simulink model "oven"  (Simulink 7.4)
settings: Solver=ode45  StartTime=0.0  StopTime=1000  MaxStep=0.1  RelTol=1e-3
undefined symbols (not defined in the file): slDataTypeAndScale
libraries: simulink x1
settings Model: Creator=psonna  LastModifiedBy=psonna

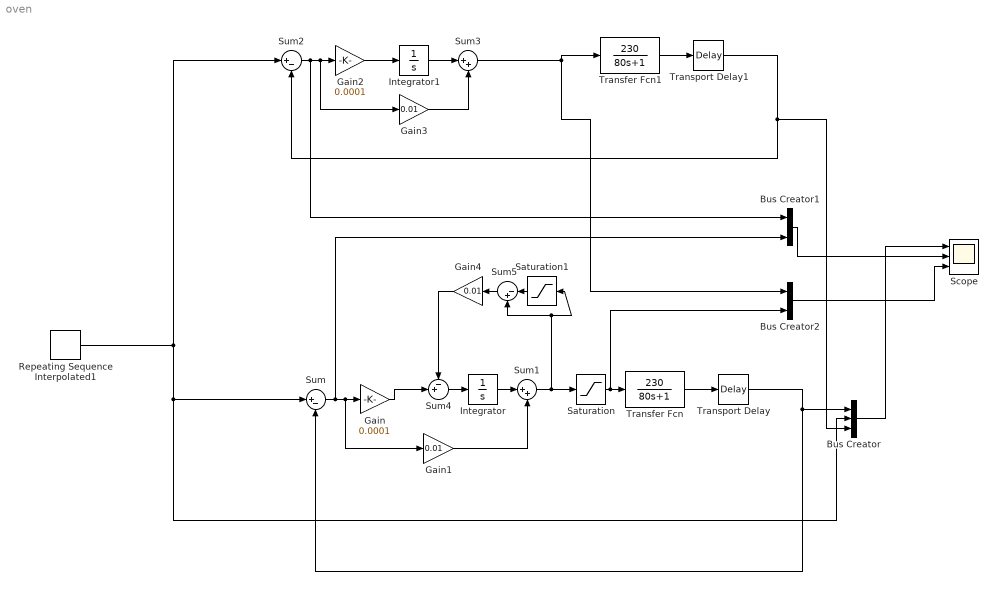
== system oven ==
  Bus Creator : BusCreator  Inputs=3
  Bus Creator1 : BusCreator  Inputs=2
  Bus Creator2 : BusCreator  Inputs=2
  Gain : Gain  Gain=0.0001  ParameterDataType=fixdt(1, 16)  ParameterScaling=2^0  OutDataType=fixdt(1, 16)  OutScaling=2^0
  Gain1 : Gain  Gain=0.01  ParameterDataType=fixdt(1, 16)  ParameterScaling=2^0  OutDataType=fixdt(1, 16)  OutScaling=2^0
  Gain2 : Gain  Gain=0.0001  ParameterDataType=fixdt(1, 16)  ParameterScaling=2^0  OutDataType=fixdt(1, 16)  OutScaling=2^0
  Gain3 : Gain  Gain=0.01  ParameterDataType=fixdt(1, 16)  ParameterScaling=2^0  OutDataType=fixdt(1, 16)  OutScaling=2^0
  Gain4 : Gain  Gain=0.01  ParameterDataType=fixdt(1, 16)  ParameterScaling=2^0  OutDataType=fixdt(1, 16)  OutScaling=2^0
  Integrator : Integrator
  Integrator1 : Integrator
  Repeating Sequence Interpolated1 : simulink/Sources/Repeating Sequence Interpolated  SystemSampleTime=-1  OutValues=[25 150 180 210 180 25 25].'  TimeValues=[0 90 180 210 240 300 1000].'  LookUpMeth=Interpolation-Use End Values  tsamp=0.01  OutMin=[]  OutMax=[]  OutDataTypeStr=double  OutputDataTypeScalingMode=double  OutDataType=slDataTypeAndScale(('double'),('2^(-10)'))  OutScaling=[]
  Saturation : Saturate  UpperLimit=1  LowerLimit=0  OutDataType=fixdt(1, 16)  OutScaling=2^0
  Saturation1 : Saturate  UpperLimit=1  LowerLimit=0  OutDataType=fixdt(1, 16)  OutScaling=2^0
  Scope : Scope  NumInputPorts=3
      settings: YMin=0~-5~-5  YMax=225~5~5
  Sum : Sum  Inputs=|+-  OutDataType=fixdt(1, 16)  OutScaling=2^0
  Sum1 : Sum  Inputs=|++  OutDataType=fixdt(1, 16)  OutScaling=2^0
  Sum2 : Sum  Inputs=|+-  OutDataType=fixdt(1, 16)  OutScaling=2^0
  Sum3 : Sum  Inputs=|++  OutDataType=fixdt(1, 16)  OutScaling=2^0
  Sum4 : Sum  Inputs=-+|  OutDataType=fixdt(1, 16)  OutScaling=2^0
  Sum5 : Sum  Inputs=|-+  OutDataType=fixdt(1, 16)  OutScaling=2^0
  Transfer Fcn : TransferFcn  Numerator=[230]  Denominator=[80 1]
  Transfer Fcn1 : TransferFcn  Numerator=[230]  Denominator=[80 1]
  Transport Delay : TransportDelay  DelayTime=10
  Transport Delay1 : TransportDelay  DelayTime=10
  wires:
  Transfer Fcn/1 -> Transport Delay/1
  Bus Creator/1 -> Scope/1
  Transport Delay/1 -> Sum/2, Bus Creator/1
  Sum/1 -> Gain/1, Gain1/1, Bus Creator1/2
  Integrator/1 -> Sum1/1
  Sum1/1 -> Saturation/1, Sum5/2, Saturation1/1
  Gain1/1 -> Sum1/2
  Saturation/1 -> Transfer Fcn/1, Bus Creator2/2
  Transfer Fcn1/1 -> Transport Delay1/1
  Transport Delay1/1 -> Sum2/2, Bus Creator/3
  Sum2/1 -> Gain2/1, Gain3/1, Bus Creator1/1
  Gain2/1 -> Integrator1/1
  Integrator1/1 -> Sum3/1
  Sum3/1 -> Bus Creator2/1, Transfer Fcn1/1
  Gain3/1 -> Sum3/2
  Bus Creator1/1 -> Scope/2
  Sum4/1 -> Integrator/1
  Gain/1 -> Sum4/2
  Saturation1/1 -> Sum5/1
  Sum5/1 -> Gain4/1
  Gain4/1 -> Sum4/1
  Bus Creator2/1 -> Scope/3
  Repeating Sequence Interpolated1/1 -> Sum2/1, Sum/1, Bus Creator/2
